simulink library "BMS"  (R2024a)
settings: Solver=VariableStepAuto  StartTime=0.0  StopTime=10.0  RelTol=1e-3
undefined symbols (not defined in the file or in its folder): raptor_xcp_function
libraries: Raptor_lib x8
settings Model: Creator=serga  LastModifiedBy=msufs

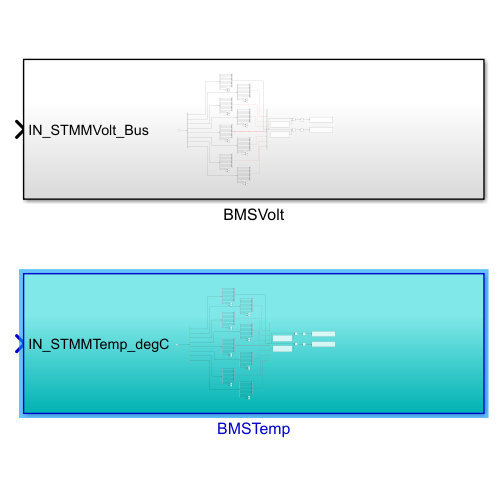
[thumbnail: Simulink's stored preview of the top-level diagram]
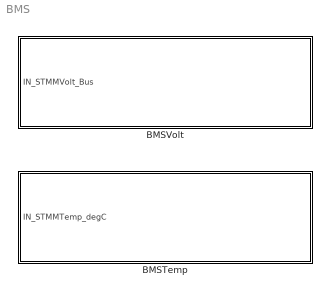
== system BMS ==
  BMSTemp : Subsystem
  BMSVolt : Subsystem

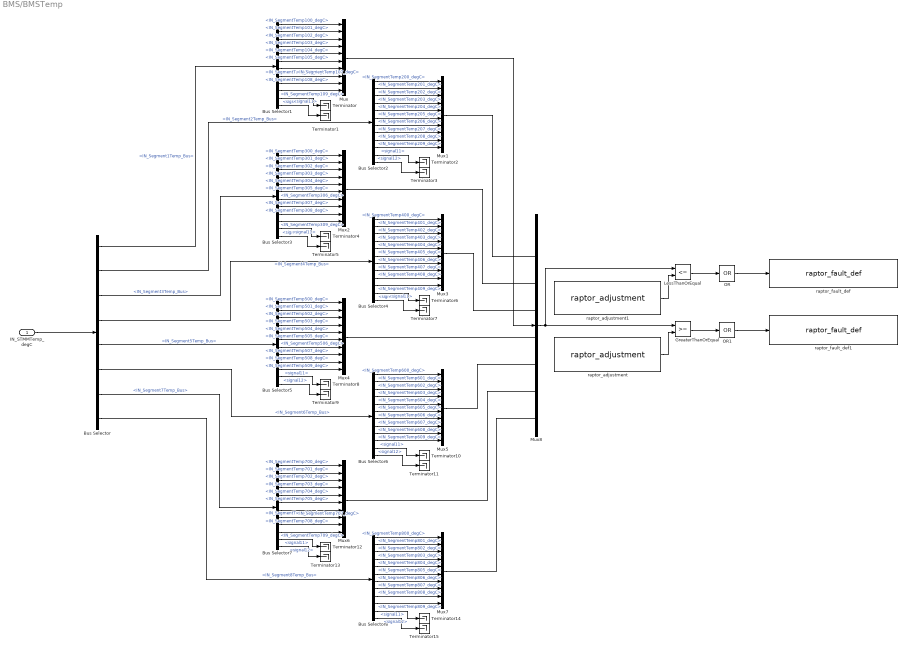
== system BMS/BMSTemp ==
  IN_STMMTemp_degC : Inport
  Bus Selector : BusSelector  OutputSignals=IN_Segment1Temp_Bus,IN_Segment2Temp_Bus,IN_Segment3Temp_Bus,IN_Segment4Temp_Bus,IN_Segment5Temp_Bus,IN_Segment6Temp_Bus,IN_Segment7Temp_Bus,IN_Segment8Temp_Bus
  Bus Selector1 : BusSelector  OutputSignals=IN_SegmentTemp100_degC,IN_SegmentTemp101_degC,IN_SegmentTemp102_degC,IN_SegmentTemp103_degC,IN_SegmentTemp104_degC,IN_SegmentTemp105_degC,IN_SegmentTemp106_degC,IN_SegmentTemp107_degC,IN_SegmentTemp108_degC,IN_SegmentTemp109_degC,signal11,signal12
  Bus Selector2 : BusSelector  OutputSignals=IN_SegmentTemp200_degC,IN_SegmentTemp201_degC,IN_SegmentTemp202_degC,IN_SegmentTemp203_degC,IN_SegmentTemp204_degC,IN_SegmentTemp205_degC,IN_SegmentTemp206_degC,IN_SegmentTemp207_degC,IN_SegmentTemp208_degC,IN_SegmentTemp209_degC,signal11,signal12
  Bus Selector3 : BusSelector  OutputSignals=IN_SegmentTemp300_degC,IN_SegmentTemp301_degC,IN_SegmentTemp302_degC,IN_SegmentTemp303_degC,IN_SegmentTemp304_degC,IN_SegmentTemp305_degC,IN_SegmentTemp306_degC,IN_SegmentTemp307_degC,IN_SegmentTemp308_degC,IN_SegmentTemp309_degC,signal11,signal12
  Bus Selector4 : BusSelector  OutputSignals=IN_SegmentTemp400_degC,IN_SegmentTemp401_degC,IN_SegmentTemp402_degC,IN_SegmentTemp403_degC,IN_SegmentTemp404_degC,IN_SegmentTemp405_degC,IN_SegmentTemp406_degC,IN_SegmentTemp407_degC,IN_SegmentTemp408_degC,IN_SegmentTemp409_degC,signal11,signal12
  Bus Selector5 : BusSelector  OutputSignals=IN_SegmentTemp500_degC,IN_SegmentTemp501_degC,IN_SegmentTemp502_degC,IN_SegmentTemp503_degC,IN_SegmentTemp504_degC,IN_SegmentTemp505_degC,IN_SegmentTemp506_degC,IN_SegmentTemp507_degC,IN_SegmentTemp508_degC,IN_SegmentTemp509_degC,signal11,signal12
  Bus Selector6 : BusSelector  OutputSignals=IN_SegmentTemp600_degC,IN_SegmentTemp601_degC,IN_SegmentTemp602_degC,IN_SegmentTemp603_degC,IN_SegmentTemp604_degC,IN_SegmentTemp605_degC,IN_SegmentTemp606_degC,IN_SegmentTemp607_degC,IN_SegmentTemp608_degC,IN_SegmentTemp609_degC,signal11,signal12
  Bus Selector7 : BusSelector  OutputSignals=IN_SegmentTemp700_degC,IN_SegmentTemp701_degC,IN_SegmentTemp702_degC,IN_SegmentTemp703_degC,IN_SegmentTemp704_degC,IN_SegmentTemp705_degC,IN_SegmentTemp706_degC,IN_SegmentTemp707_degC,IN_SegmentTemp708_degC,IN_SegmentTemp709_degC,signal11,signal12
  Bus Selector8 : BusSelector  OutputSignals=IN_SegmentTemp800_degC,IN_SegmentTemp801_degC,IN_SegmentTemp802_degC,IN_SegmentTemp803_degC,IN_SegmentTemp804_degC,IN_SegmentTemp805_degC,IN_SegmentTemp806_degC,IN_SegmentTemp807_degC,IN_SegmentTemp808_degC,IN_SegmentTemp809_degC,signal11,signal12
  GreaterThanOrEqual : RelationalOperator  OutDataTypeStr=boolean  RndMeth=Simplest  InputSameDT=off
  LessThanOrEqual : RelationalOperator  Operator=<=  OutDataTypeStr=boolean  RndMeth=Simplest  InputSameDT=off
  Mux{,1..7} (8 alike) : Mux  Inputs=10
  Mux8 : Mux  Inputs=1
  OR : Logic  Operator=OR  Inputs=1  AllPortsSameDT=off  OutDataTypeStr=boolean
  OR1 : Logic  Operator=OR  Inputs=1  AllPortsSameDT=off  OutDataTypeStr=boolean
  Terminator{,1..15} (16 alike) : Terminator
  raptor_adjustment : Raptor_lib/Data Storage/raptor_adjustment  paramName='CTRL_SegmentOverTempThresh_degC'  nameSource=Parameter  initValue=50  dataType=single  storage=Calibration  calDispType=Number  calEnum={'False', 'True'}  calGain=1.0  calOffset=0.0  calMax=inf  calMin=-inf  calFormat='-1'  calUnit=''  calHelp=''  calAccess=1  calFunction=raptor_xcp_function(gcb)  calDispHeaders=off  calColHeaders={'Col1' 'Col2' 'Col3'}  calRowHeaders={'Row1' 'Row2' 'Row3'}
      settings: SourceProductName=Raptor
  raptor_adjustment1 : Raptor_lib/Data Storage/raptor_adjustment  paramName='CTRL_SegmentUnderTempThresh_degC'  nameSource=Parameter  initValue=-10  dataType=single  storage=Calibration  calDispType=Number  calEnum={'False', 'True'}  calGain=1.0  calOffset=0.0  calMax=inf  calMin=-inf  calFormat='-1'  calUnit=''  calHelp=''  calAccess=1  calFunction=raptor_xcp_function(gcb)  calDispHeaders=off  calColHeaders={'Col1' 'Col2' 'Col3'}  calRowHeaders={'Row1' 'Row2' 'Row3'}
      settings: SourceProductName=Raptor
  raptor_fault_def : Raptor_lib/Faults/raptor_fault_def  faultName='CTRL_SegmentUnderTempFault'  persist=on  sticky=off  emisRelated=off  singleTrip=off  clearMethod=Standard  xLimit=25  yLimit=50  calEnable=on  addDisable=off  calAccess=1  calFunction='System | FaultManager'
      settings: SourceProductName=Raptor
  raptor_fault_def1 : Raptor_lib/Faults/raptor_fault_def  faultName='CTRL_SegmentOverTempFault'  persist=on  sticky=off  emisRelated=off  singleTrip=off  clearMethod=Standard  xLimit=25  yLimit=50  calEnable=on  addDisable=off  calAccess=1  calFunction='System | FaultManager'
      settings: SourceProductName=Raptor
  wires:
  IN_STMMTemp_degC/1 -> Bus Selector/1
  Bus Selector7/3 -> Mux6/3  "<IN_SegmentTemp702_degC>"
  Bus Selector2/5 -> Mux1/5  "<IN_SegmentTemp204_degC>"
  Bus Selector7/10 -> Mux6/10  "<IN_SegmentTemp709_degC>"
  Bus Selector1/7 -> Mux/7  "<IN_SegmentTemp106_degC>"
  Bus Selector5/2 -> Mux4/2  "<IN_SegmentTemp501_degC>"
  Bus Selector1/10 -> Mux/10  "<IN_SegmentTemp109_degC>"
  Bus Selector1/6 -> Mux/6  "<IN_SegmentTemp105_degC>"
  Bus Selector5/11 -> Terminator8/1  "<signal11>"
  Bus Selector7/1 -> Mux6/1  "<IN_SegmentTemp700_degC>"
  Bus Selector4/2 -> Mux3/2  "<IN_SegmentTemp401_degC>"
  Bus Selector/1 -> Bus Selector1/1  "<IN_Segment1Temp_Bus>"
  Bus Selector2/4 -> Mux1/4  "<IN_SegmentTemp203_degC>"
  Bus Selector7/2 -> Mux6/2  "<IN_SegmentTemp701_degC>"
  Bus Selector1/5 -> Mux/5  "<IN_SegmentTemp104_degC>"
  Bus Selector8/5 -> Mux7/5  "<IN_SegmentTemp804_degC>"
  Bus Selector4/3 -> Mux3/3  "<IN_SegmentTemp402_degC>"
  Bus Selector1/2 -> Mux/2  "<IN_SegmentTemp101_degC>"
  Bus Selector4/4 -> Mux3/4  "<IN_SegmentTemp403_degC>"
  Bus Selector6/9 -> Mux5/9  "<IN_SegmentTemp608_degC>"
  Bus Selector3/4 -> Mux2/4  "<IN_SegmentTemp303_degC>"
  Bus Selector1/4 -> Mux/4  "<IN_SegmentTemp103_degC>"
  Bus Selector7/4 -> Mux6/4  "<IN_SegmentTemp703_degC>"
  Bus Selector5/12 -> Terminator9/1  "<signal12>"
  Bus Selector6/4 -> Mux5/4  "<IN_SegmentTemp603_degC>"
  Bus Selector5/10 -> Mux4/10  "<IN_SegmentTemp509_degC>"
  Bus Selector5/5 -> Mux4/5  "<IN_SegmentTemp504_degC>"
  Bus Selector3/1 -> Mux2/1  "<IN_SegmentTemp300_degC>"
  Bus Selector6/5 -> Mux5/5  "<IN_SegmentTemp604_degC>"
  Mux6/1 -> ?
  Bus Selector3/8 -> Mux2/8  "<IN_SegmentTemp307_degC>"
  Bus Selector2/9 -> Mux1/9  "<IN_SegmentTemp208_degC>"
  Bus Selector5/6 -> Mux4/6  "<IN_SegmentTemp505_degC>"
  Bus Selector1/12 -> Terminator1/1  "<signal12>"
  Bus Selector2/6 -> Mux1/6  "<IN_SegmentTemp205_degC>"
  Bus Selector2/3 -> Mux1/3  "<IN_SegmentTemp202_degC>"
  Bus Selector/7 -> Bus Selector7/1  "<IN_Segment7Temp_Bus>"
  Bus Selector7/7 -> Mux6/7  "<IN_SegmentTemp706_degC>"
  Bus Selector2/8 -> Mux1/8  "<IN_SegmentTemp207_degC>"
  Bus Selector7/9 -> Mux6/9  "<IN_SegmentTemp708_degC>"
  Bus Selector/6 -> Bus Selector6/1  "<IN_Segment6Temp_Bus>"
  Bus Selector7/11 -> Terminator12/1  "<signal11>"
  Bus Selector4/5 -> Mux3/5  "<IN_SegmentTemp404_degC>"
  Bus Selector3/6 -> Mux2/6  "<IN_SegmentTemp305_degC>"
  Bus Selector3/7 -> Mux2/7  "<IN_SegmentTemp306_degC>"
  Bus Selector3/9 -> Mux2/9  "<IN_SegmentTemp308_degC>"
  Bus Selector3/12 -> Terminator5/1  "<signal12>"
  Bus Selector3/10 -> Mux2/10  "<IN_SegmentTemp309_degC>"
  Bus Selector4/1 -> Mux3/1  "<IN_SegmentTemp400_degC>"
  Bus Selector2/1 -> Mux1/1  "<IN_SegmentTemp200_degC>"
  Bus Selector2/7 -> Mux1/7  "<IN_SegmentTemp206_degC>"
  Bus Selector6/8 -> Mux5/8  "<IN_SegmentTemp607_degC>"
  Bus Selector1/9 -> Mux/9  "<IN_SegmentTemp108_degC>"
  Bus Selector2/12 -> Terminator3/1  "<signal12>"
  Bus Selector3/2 -> Mux2/2  "<IN_SegmentTemp301_degC>"
  Bus Selector/3 -> Bus Selector3/1  "<IN_Segment3Temp_Bus>"
  Bus Selector6/6 -> Mux5/6  "<IN_SegmentTemp605_degC>"
  Bus Selector5/8 -> Mux4/8  "<IN_SegmentTemp507_degC>"
  Bus Selector/4 -> Bus Selector4/1  "<IN_Segment4Temp_Bus>"
  Bus Selector5/7 -> Mux4/7  "<IN_SegmentTemp506_degC>"
  Bus Selector7/12 -> Terminator13/1  "<signal12>"
  Bus Selector5/9 -> Mux4/9  "<IN_SegmentTemp508_degC>"
  Bus Selector4/7 -> Mux3/7  "<IN_SegmentTemp406_degC>"
  Bus Selector6/7 -> Mux5/7  "<IN_SegmentTemp606_degC>"
  Bus Selector1/3 -> Mux/3  "<IN_SegmentTemp102_degC>"
  Bus Selector1/8 -> Mux/8  "<IN_SegmentTemp107_degC>"
  Bus Selector1/1 -> Mux/1  "<IN_SegmentTemp100_degC>"
  Bus Selector3/3 -> Mux2/3  "<IN_SegmentTemp302_degC>"
  Bus Selector2/11 -> Terminator2/1  "<signal11>"
  Bus Selector4/10 -> Mux3/10  "<IN_SegmentTemp409_degC>"
  Bus Selector4/12 -> Terminator7/1  "<signal12>"
  Bus Selector/5 -> Bus Selector5/1  "<IN_Segment5Temp_Bus>"
  Bus Selector2/2 -> Mux1/2  "<IN_SegmentTemp201_degC>"
  Bus Selector4/8 -> Mux3/8  "<IN_SegmentTemp407_degC>"
  OR1/1 -> raptor_fault_def1/1
  Bus Selector1/11 -> Terminator/1  "<signal11>"
  Bus Selector8/2 -> Mux7/2  "<IN_SegmentTemp801_degC>"
  Bus Selector/8 -> Bus Selector8/1  "<IN_Segment8Temp_Bus>"
  Bus Selector8/3 -> Mux7/3  "<IN_SegmentTemp802_degC>"
  Mux1/1 -> ?
  Bus Selector4/9 -> Mux3/9  "<IN_SegmentTemp408_degC>"
  Bus Selector8/10 -> Mux7/10  "<IN_SegmentTemp809_degC>"
  Bus Selector5/1 -> Mux4/1  "<IN_SegmentTemp500_degC>"
  Bus Selector3/11 -> Terminator4/1  "<signal11>"
  Bus Selector8/6 -> Mux7/6  "<IN_SegmentTemp805_degC>"
  Bus Selector6/1 -> Mux5/1  "<IN_SegmentTemp600_degC>"
  Bus Selector8/11 -> Terminator14/1  "<signal11>"
  Bus Selector5/4 -> Mux4/4  "<IN_SegmentTemp503_degC>"
  Bus Selector3/5 -> Mux2/5  "<IN_SegmentTemp304_degC>"
  Bus Selector2/10 -> Mux1/10  "<IN_SegmentTemp209_degC>"
  Bus Selector7/8 -> Mux6/8  "<IN_SegmentTemp707_degC>"
  Bus Selector4/11 -> Terminator6/1  "<signal11>"
  Bus Selector5/3 -> Mux4/3  "<IN_SegmentTemp502_degC>"
  Bus Selector8/7 -> Mux7/7  "<IN_SegmentTemp806_degC>"
  Bus Selector8/9 -> Mux7/9  "<IN_SegmentTemp808_degC>"
  Bus Selector7/5 -> Mux6/5  "<IN_SegmentTemp704_degC>"
  Mux4/1 -> ?
  Bus Selector/2 -> Bus Selector2/1  "<IN_Segment2Temp_Bus>"
  Bus Selector8/12 -> Terminator15/1  "<signal12>"
  GreaterThanOrEqual/1 -> OR1/1
  Bus Selector6/11 -> Terminator10/1  "<signal11>"
  Mux7/1 -> ?
  Mux5/1 -> ?
  Bus Selector6/10 -> Mux5/10  "<IN_SegmentTemp609_degC>"
  Mux8/1 -> LessThanOrEqual/1, GreaterThanOrEqual/1
  Bus Selector7/6 -> Mux6/6  "<IN_SegmentTemp705_degC>"
  Bus Selector6/3 -> Mux5/3  "<IN_SegmentTemp602_degC>"
  Mux2/1 -> ?
  Bus Selector8/8 -> Mux7/8  "<IN_SegmentTemp807_degC>"
  raptor_adjustment1/1 -> LessThanOrEqual/2
  Bus Selector6/2 -> Mux5/2  "<IN_SegmentTemp601_degC>"
  Bus Selector8/1 -> Mux7/1  "<IN_SegmentTemp800_degC>"
  LessThanOrEqual/1 -> OR/1
  Mux3/1 -> ?
  Bus Selector6/12 -> Terminator11/1  "<signal12>"
  raptor_adjustment/1 -> GreaterThanOrEqual/2
  Mux/1 -> Mux8/1
  OR/1 -> raptor_fault_def/1
  Bus Selector8/4 -> Mux7/4  "<IN_SegmentTemp803_degC>"
  Bus Selector4/6 -> Mux3/6  "<IN_SegmentTemp405_degC>"

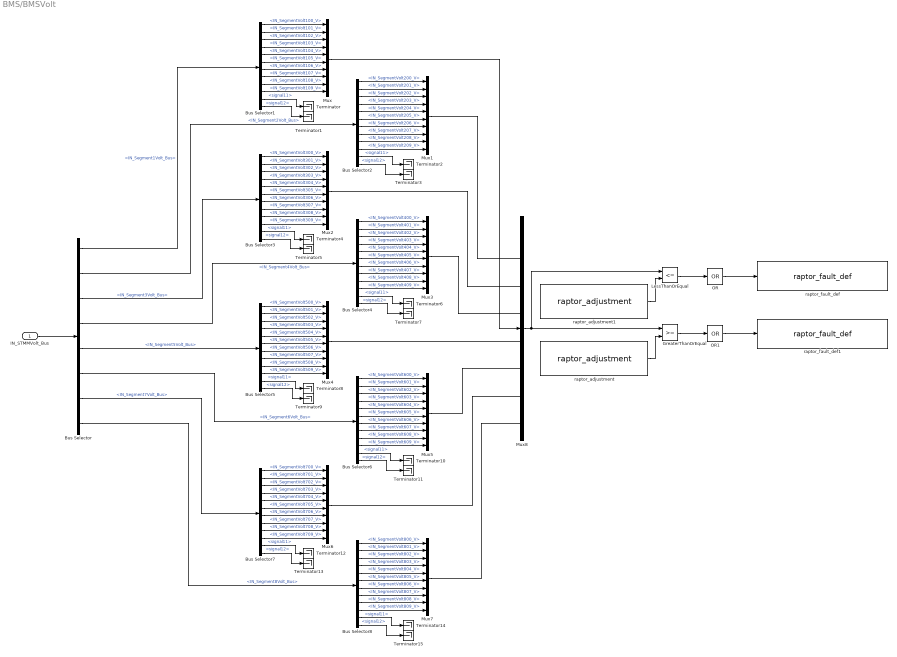
== system BMS/BMSVolt ==
  IN_STMMVolt_Bus : Inport
  Bus Selector : BusSelector  OutputSignals=IN_Segment1Volt_Bus,IN_Segment2Volt_Bus,IN_Segment3Volt_Bus,IN_Segment4Volt_Bus,IN_Segment5Volt_Bus,IN_Segment6Volt_Bus,IN_Segment7Volt_Bus,IN_Segment8Volt_Bus
  Bus Selector1 : BusSelector  OutputSignals=IN_SegmentVolt100_V,IN_SegmentVolt101_V,IN_SegmentVolt102_V,IN_SegmentVolt103_V,IN_SegmentVolt104_V,IN_SegmentVolt105_V,IN_SegmentVolt106_V,IN_SegmentVolt107_V,IN_SegmentVolt108_V,IN_SegmentVolt109_V,signal11,signal12
  Bus Selector2 : BusSelector  OutputSignals=IN_SegmentVolt200_V,IN_SegmentVolt201_V,IN_SegmentVolt202_V,IN_SegmentVolt203_V,IN_SegmentVolt204_V,IN_SegmentVolt205_V,IN_SegmentVolt206_V,IN_SegmentVolt207_V,IN_SegmentVolt208_V,IN_SegmentVolt209_V,signal11,signal12
  Bus Selector3 : BusSelector  OutputSignals=IN_SegmentVolt300_V,IN_SegmentVolt301_V,IN_SegmentVolt302_V,IN_SegmentVolt303_V,IN_SegmentVolt304_V,IN_SegmentVolt305_V,IN_SegmentVolt306_V,IN_SegmentVolt307_V,IN_SegmentVolt308_V,IN_SegmentVolt309_V,signal11,signal12
  Bus Selector4 : BusSelector  OutputSignals=IN_SegmentVolt400_V,IN_SegmentVolt401_V,IN_SegmentVolt402_V,IN_SegmentVolt403_V,IN_SegmentVolt404_V,IN_SegmentVolt405_V,IN_SegmentVolt406_V,IN_SegmentVolt407_V,IN_SegmentVolt408_V,IN_SegmentVolt409_V,signal11,signal12
  Bus Selector5 : BusSelector  OutputSignals=IN_SegmentVolt500_V,IN_SegmentVolt501_V,IN_SegmentVolt502_V,IN_SegmentVolt503_V,IN_SegmentVolt504_V,IN_SegmentVolt505_V,IN_SegmentVolt506_V,IN_SegmentVolt507_V,IN_SegmentVolt508_V,IN_SegmentVolt509_V,signal11,signal12
  Bus Selector6 : BusSelector  OutputSignals=IN_SegmentVolt600_V,IN_SegmentVolt601_V,IN_SegmentVolt602_V,IN_SegmentVolt603_V,IN_SegmentVolt604_V,IN_SegmentVolt605_V,IN_SegmentVolt606_V,IN_SegmentVolt607_V,IN_SegmentVolt608_V,IN_SegmentVolt609_V,signal11,signal12
  Bus Selector7 : BusSelector  OutputSignals=IN_SegmentVolt700_V,IN_SegmentVolt701_V,IN_SegmentVolt702_V,IN_SegmentVolt703_V,IN_SegmentVolt704_V,IN_SegmentVolt705_V,IN_SegmentVolt706_V,IN_SegmentVolt707_V,IN_SegmentVolt708_V,IN_SegmentVolt709_V,signal11,signal12
  Bus Selector8 : BusSelector  OutputSignals=IN_SegmentVolt800_V,IN_SegmentVolt801_V,IN_SegmentVolt802_V,IN_SegmentVolt803_V,IN_SegmentVolt804_V,IN_SegmentVolt805_V,IN_SegmentVolt806_V,IN_SegmentVolt807_V,IN_SegmentVolt808_V,IN_SegmentVolt809_V,signal11,signal12
  GreaterThanOrEqual : RelationalOperator  OutDataTypeStr=boolean  RndMeth=Simplest  InputSameDT=off
  LessThanOrEqual : RelationalOperator  Operator=<=  OutDataTypeStr=boolean  RndMeth=Simplest  InputSameDT=off
  Mux{,1..7} (8 alike) : Mux  Inputs=10
  Mux8 : Mux  Inputs=1
  OR : Logic  Operator=OR  Inputs=1  AllPortsSameDT=off  OutDataTypeStr=boolean
  OR1 : Logic  Operator=OR  Inputs=1  AllPortsSameDT=off  OutDataTypeStr=boolean
  Terminator{,1..15} (16 alike) : Terminator
  raptor_adjustment : Raptor_lib/Data Storage/raptor_adjustment  paramName='CTRL_SegmentOverVoltThresh_V'  nameSource=Parameter  initValue=4.2  dataType=single  storage=Calibration  calDispType=Number  calEnum={'False', 'True'}  calGain=1.0  calOffset=0.0  calMax=inf  calMin=-inf  calFormat='-1'  calUnit=''  calHelp=''  calAccess=1  calFunction=raptor_xcp_function(gcb)  calDispHeaders=off  calColHeaders={'Col1' 'Col2' 'Col3'}  calRowHeaders={'Row1' 'Row2' 'Row3'}
      settings: SourceProductName=Raptor
  raptor_adjustment1 : Raptor_lib/Data Storage/raptor_adjustment  paramName='CTRL_SegmentUnderVoltThresh_V'  nameSource=Parameter  initValue=2.7  dataType=single  storage=Calibration  calDispType=Number  calEnum={'False', 'True'}  calGain=1.0  calOffset=0.0  calMax=inf  calMin=-inf  calFormat='-1'  calUnit=''  calHelp=''  calAccess=1  calFunction=raptor_xcp_function(gcb)  calDispHeaders=off  calColHeaders={'Col1' 'Col2' 'Col3'}  calRowHeaders={'Row1' 'Row2' 'Row3'}
      settings: SourceProductName=Raptor
  raptor_fault_def : Raptor_lib/Faults/raptor_fault_def  faultName='CTRL_SegmentUnderVoltFault'  persist=on  sticky=off  emisRelated=off  singleTrip=off  clearMethod=Standard  xLimit=25  yLimit=50  calEnable=on  addDisable=off  calAccess=1  calFunction='System | FaultManager'
      settings: SourceProductName=Raptor
  raptor_fault_def1 : Raptor_lib/Faults/raptor_fault_def  faultName='CTRL_SegmentOverVoltFault'  persist=on  sticky=off  emisRelated=off  singleTrip=off  clearMethod=Standard  xLimit=25  yLimit=50  calEnable=on  addDisable=off  calAccess=1  calFunction='System | FaultManager'
      settings: SourceProductName=Raptor
  wires:
  GreaterThanOrEqual/1 -> OR1/1
  LessThanOrEqual/1 -> OR/1
  raptor_adjustment1/1 -> LessThanOrEqual/2
  raptor_adjustment/1 -> GreaterThanOrEqual/2
  Mux8/1 -> LessThanOrEqual/1, GreaterThanOrEqual/1
  Mux7/1 -> ?
  Mux6/1 -> ?
  Mux5/1 -> ?
  Mux4/1 -> ?
  Mux3/1 -> ?
  Mux2/1 -> ?
  Mux1/1 -> ?
  Mux/1 -> Mux8/1
  Bus Selector8/12 -> Terminator15/1  "<signal12>"
  Bus Selector8/11 -> Terminator14/1  "<signal11>"
  Bus Selector8/10 -> Mux7/10  "<IN_SegmentVolt809_V>"
  Bus Selector8/9 -> Mux7/9  "<IN_SegmentVolt808_V>"
  Bus Selector8/8 -> Mux7/8  "<IN_SegmentVolt807_V>"
  Bus Selector8/7 -> Mux7/7  "<IN_SegmentVolt806_V>"
  Bus Selector8/6 -> Mux7/6  "<IN_SegmentVolt805_V>"
  Bus Selector8/5 -> Mux7/5  "<IN_SegmentVolt804_V>"
  Bus Selector8/4 -> Mux7/4  "<IN_SegmentVolt803_V>"
  Bus Selector8/3 -> Mux7/3  "<IN_SegmentVolt802_V>"
  Bus Selector8/2 -> Mux7/2  "<IN_SegmentVolt801_V>"
  Bus Selector8/1 -> Mux7/1  "<IN_SegmentVolt800_V>"
  Bus Selector/8 -> Bus Selector8/1  "<IN_Segment8Volt_Bus>"
  Bus Selector7/12 -> Terminator13/1  "<signal12>"
  Bus Selector7/11 -> Terminator12/1  "<signal11>"
  Bus Selector7/10 -> Mux6/10  "<IN_SegmentVolt709_V>"
  Bus Selector7/9 -> Mux6/9  "<IN_SegmentVolt708_V>"
  Bus Selector7/8 -> Mux6/8  "<IN_SegmentVolt707_V>"
  Bus Selector7/7 -> Mux6/7  "<IN_SegmentVolt706_V>"
  Bus Selector7/6 -> Mux6/6  "<IN_SegmentVolt705_V>"
  Bus Selector7/5 -> Mux6/5  "<IN_SegmentVolt704_V>"
  Bus Selector7/4 -> Mux6/4  "<IN_SegmentVolt703_V>"
  Bus Selector7/3 -> Mux6/3  "<IN_SegmentVolt702_V>"
  Bus Selector7/2 -> Mux6/2  "<IN_SegmentVolt701_V>"
  Bus Selector7/1 -> Mux6/1  "<IN_SegmentVolt700_V>"
  Bus Selector/7 -> Bus Selector7/1  "<IN_Segment7Volt_Bus>"
  Bus Selector6/12 -> Terminator11/1  "<signal12>"
  Bus Selector6/11 -> Terminator10/1  "<signal11>"
  Bus Selector6/10 -> Mux5/10  "<IN_SegmentVolt609_V>"
  Bus Selector6/9 -> Mux5/9  "<IN_SegmentVolt608_V>"
  Bus Selector6/8 -> Mux5/8  "<IN_SegmentVolt607_V>"
  Bus Selector6/7 -> Mux5/7  "<IN_SegmentVolt606_V>"
  Bus Selector6/6 -> Mux5/6  "<IN_SegmentVolt605_V>"
  Bus Selector6/5 -> Mux5/5  "<IN_SegmentVolt604_V>"
  Bus Selector6/4 -> Mux5/4  "<IN_SegmentVolt603_V>"
  Bus Selector6/3 -> Mux5/3  "<IN_SegmentVolt602_V>"
  Bus Selector6/2 -> Mux5/2  "<IN_SegmentVolt601_V>"
  Bus Selector6/1 -> Mux5/1  "<IN_SegmentVolt600_V>"
  Bus Selector/6 -> Bus Selector6/1  "<IN_Segment6Volt_Bus>"
  Bus Selector5/12 -> Terminator9/1  "<signal12>"
  Bus Selector5/11 -> Terminator8/1  "<signal11>"
  Bus Selector5/10 -> Mux4/10  "<IN_SegmentVolt509_V>"
  Bus Selector5/9 -> Mux4/9  "<IN_SegmentVolt508_V>"
  Bus Selector5/7 -> Mux4/7  "<IN_SegmentVolt506_V>"
  Bus Selector5/8 -> Mux4/8  "<IN_SegmentVolt507_V>"
  Bus Selector5/6 -> Mux4/6  "<IN_SegmentVolt505_V>"
  Bus Selector5/5 -> Mux4/5  "<IN_SegmentVolt504_V>"
  Bus Selector5/4 -> Mux4/4  "<IN_SegmentVolt503_V>"
  Bus Selector5/3 -> Mux4/3  "<IN_SegmentVolt502_V>"
  Bus Selector5/2 -> Mux4/2  "<IN_SegmentVolt501_V>"
  Bus Selector5/1 -> Mux4/1  "<IN_SegmentVolt500_V>"
  Bus Selector/5 -> Bus Selector5/1  "<IN_Segment5Volt_Bus>"
  Bus Selector4/12 -> Terminator7/1  "<signal12>"
  Bus Selector4/11 -> Terminator6/1  "<signal11>"
  Bus Selector4/10 -> Mux3/10  "<IN_SegmentVolt409_V>"
  Bus Selector4/9 -> Mux3/9  "<IN_SegmentVolt408_V>"
  Bus Selector4/8 -> Mux3/8  "<IN_SegmentVolt407_V>"
  Bus Selector4/7 -> Mux3/7  "<IN_SegmentVolt406_V>"
  Bus Selector4/6 -> Mux3/6  "<IN_SegmentVolt405_V>"
  Bus Selector4/5 -> Mux3/5  "<IN_SegmentVolt404_V>"
  Bus Selector4/4 -> Mux3/4  "<IN_SegmentVolt403_V>"
  Bus Selector4/3 -> Mux3/3  "<IN_SegmentVolt402_V>"
  Bus Selector4/2 -> Mux3/2  "<IN_SegmentVolt401_V>"
  Bus Selector4/1 -> Mux3/1  "<IN_SegmentVolt400_V>"
  Bus Selector/4 -> Bus Selector4/1  "<IN_Segment4Volt_Bus>"
  Bus Selector3/12 -> Terminator5/1  "<signal12>"
  Bus Selector3/11 -> Terminator4/1  "<signal11>"
  Bus Selector3/10 -> Mux2/10  "<IN_SegmentVolt309_V>"
  Bus Selector3/9 -> Mux2/9  "<IN_SegmentVolt308_V>"
  Bus Selector3/7 -> Mux2/7  "<IN_SegmentVolt306_V>"
  Bus Selector3/8 -> Mux2/8  "<IN_SegmentVolt307_V>"
  Bus Selector3/6 -> Mux2/6  "<IN_SegmentVolt305_V>"
  Bus Selector3/5 -> Mux2/5  "<IN_SegmentVolt304_V>"
  Bus Selector3/4 -> Mux2/4  "<IN_SegmentVolt303_V>"
  Bus Selector3/3 -> Mux2/3  "<IN_SegmentVolt302_V>"
  Bus Selector3/2 -> Mux2/2  "<IN_SegmentVolt301_V>"
  Bus Selector3/1 -> Mux2/1  "<IN_SegmentVolt300_V>"
  Bus Selector/3 -> Bus Selector3/1  "<IN_Segment3Volt_Bus>"
  Bus Selector2/12 -> Terminator3/1  "<signal12>"
  Bus Selector2/11 -> Terminator2/1  "<signal11>"
  Bus Selector2/10 -> Mux1/10  "<IN_SegmentVolt209_V>"
  Bus Selector2/9 -> Mux1/9  "<IN_SegmentVolt208_V>"
  Bus Selector2/8 -> Mux1/8  "<IN_SegmentVolt207_V>"
  Bus Selector2/7 -> Mux1/7  "<IN_SegmentVolt206_V>"
  Bus Selector2/6 -> Mux1/6  "<IN_SegmentVolt205_V>"
  Bus Selector2/5 -> Mux1/5  "<IN_SegmentVolt204_V>"
  Bus Selector2/4 -> Mux1/4  "<IN_SegmentVolt203_V>"
  Bus Selector2/3 -> Mux1/3  "<IN_SegmentVolt202_V>"
  Bus Selector2/2 -> Mux1/2  "<IN_SegmentVolt201_V>"
  Bus Selector2/1 -> Mux1/1  "<IN_SegmentVolt200_V>"
  Bus Selector/2 -> Bus Selector2/1  "<IN_Segment2Volt_Bus>"
  Bus Selector1/12 -> Terminator1/1  "<signal12>"
  Bus Selector1/11 -> Terminator/1  "<signal11>"
  Bus Selector1/10 -> Mux/10  "<IN_SegmentVolt109_V>"
  Bus Selector1/9 -> Mux/9  "<IN_SegmentVolt108_V>"
  Bus Selector1/8 -> Mux/8  "<IN_SegmentVolt107_V>"
  Bus Selector1/7 -> Mux/7  "<IN_SegmentVolt106_V>"
  Bus Selector1/6 -> Mux/6  "<IN_SegmentVolt105_V>"
  Bus Selector1/5 -> Mux/5  "<IN_SegmentVolt104_V>"
  Bus Selector1/4 -> Mux/4  "<IN_SegmentVolt103_V>"
  Bus Selector1/3 -> Mux/3  "<IN_SegmentVolt102_V>"
  Bus Selector1/2 -> Mux/2  "<IN_SegmentVolt101_V>"
  Bus Selector1/1 -> Mux/1  "<IN_SegmentVolt100_V>"
  Bus Selector/1 -> Bus Selector1/1  "<IN_Segment1Volt_Bus>"
  IN_STMMVolt_Bus/1 -> Bus Selector/1
  OR/1 -> raptor_fault_def/1
  OR1/1 -> raptor_fault_def1/1
